simulink model "temp"  (R2021b)
settings: Solver=VariableStepAuto  StartTime=0.0  StopTime=10.0  RelTol=1e-3
libraries: arduinolib x3
settings Model: Creator=fady  LastModifiedBy=fady

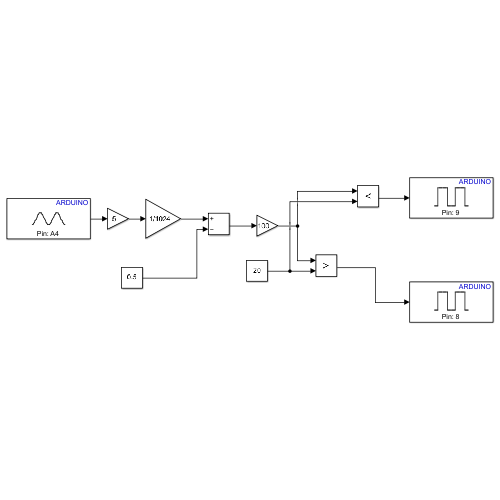
[thumbnail: Simulink's stored preview of the top-level diagram]
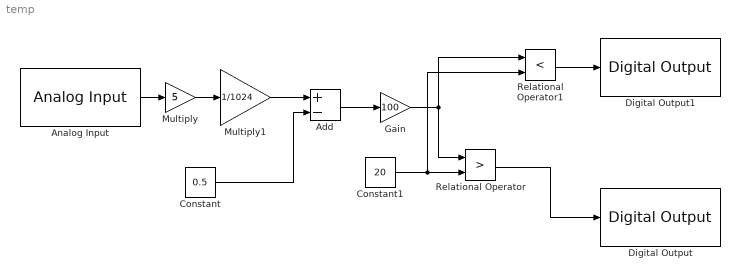
== system temp ==
  Add : Sum  Inputs=+-
  Analog Input : arduinolib/Analog Input  pinNumber=4  ReadResultsOnly=off  ConversionTriggerSource=Software  ExternalTriggerType=uint32( 0 )  OutputDataType=uint16  EnableConversionCompleteNotify=off  EnableOuputStatus=off  SampleTime=-1  blockPlatform=arduino
  Constant : Constant  Value=0.5
  Constant1 : Constant  Value=20
  Digital Output : arduinolib/Digital Output  pinNumber=8  Direction=output  blockPlatform=arduino
  Digital Output1 : arduinolib/Digital Output  pinNumber=9  Direction=output  blockPlatform=arduino
  Gain : Gain  Gain=100
  Multiply : Gain  Gain=5
  Multiply1 : Gain  Gain=1/1024
  Relational Operator : RelationalOperator  Operator=>  OutDataTypeStr=boolean  RndMeth=Simplest
  Relational Operator1 : RelationalOperator  Operator=<  OutDataTypeStr=boolean  RndMeth=Simplest
  wires:
  Analog Input/1 -> Multiply/1
  Multiply/1 -> Multiply1/1
  Multiply1/1 -> Add/1
  Constant/1 -> Add/2
  Add/1 -> Gain/1
  Gain/1 -> Relational Operator1/1, Relational Operator/1
  Constant1/1 -> Relational Operator1/2, Relational Operator/2
  Relational Operator/1 -> Digital Output/1
  Relational Operator1/1 -> Digital Output1/1
